simulink model "motor_simulink"  (R2021b)
settings: Solver=VariableStepAuto  StartTime=0.0  StopTime=1.5  MaxStep=1e-8  RelTol=1e-3
libraries: simulink x7, spsOnDelayLib x6, slpidlib x3, eePwmGeneratorTwoLevel x2, spsDCVoltageSourceLib x1, spsPermanentMagnetSynchronousMachineLib x1, spsUniversalBridgeLib x1, spsabctodq0Lib x1, spspowerguiLib x1
settings Model: SimulationMode=accelerator  Creator=phddk  LastModifiedBy=phddk
settings SolverCC: ZeroCrossAlgorithm=Adaptive

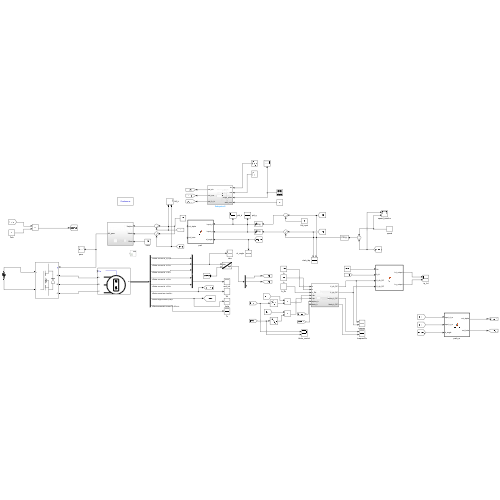
[thumbnail: Simulink's stored preview of the top-level diagram]
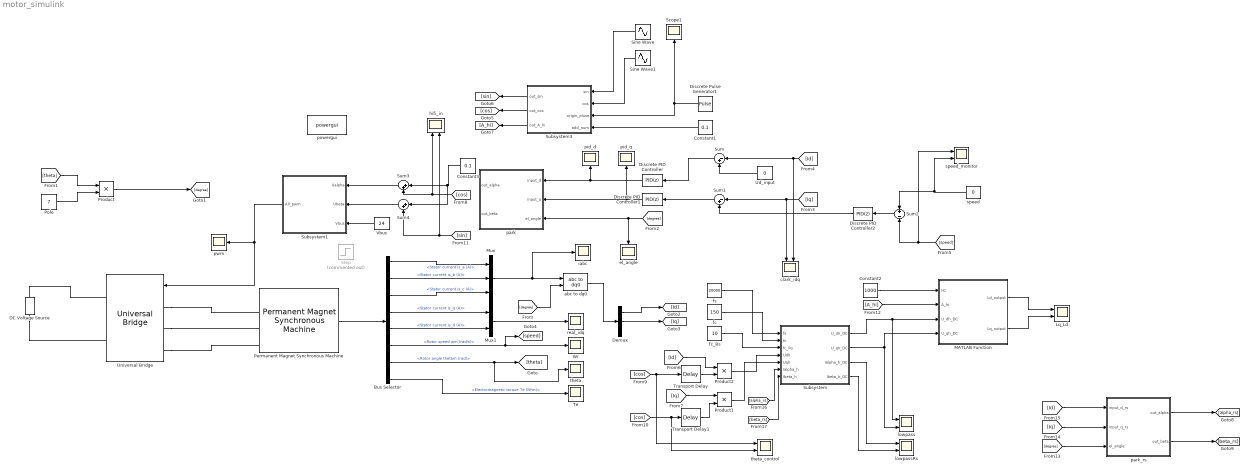
== system motor_simulink ==
  Bus Selector : BusSelector  OutputSignals=Stator current is_a (A),Stator current is_b (A),Stator current is_c (A),Stator current is_q (A),Stator current is_d (A),Rotor speed wm (rad/s),Rotor angle thetam (rad),Electromagnetic torque Te (N*m)
  Constant1 : Constant  Value=0.1
  Constant2 : Constant  Value=1000
  Constant3 : Constant  Value=0.1
  DC Voltage Source : spsDCVoltageSourceLib/DC Voltage Source  Amplitude=24  Measurements=Voltage
  Demux : Demux  Outputs=3
  Discrete Pulse Generator1 : DiscretePulseGenerator  Period=50  PulseWidth=25  SampleTime=0.001
  Discrete PID Controller : slpidlib/PID Controller  Controller=PID  Form=Parallel  TimeDomain=Discrete-time  UseExternalTs=off  SampleTime=-1  IntegratorMethod=Forward Euler  FilterMethod=Forward Euler  ControllerParametersSource=internal  P=1  I=5  D=0  UseFilter=on  N=100  TunerSelectOption=Transfer Function Based (PID Tuner App)  InitialConditionSource=internal  InitialConditionForIntegrator=0  InitialConditionForFilter=0  DifferentiatorICPrevScaledInput=0  ExternalReset=none  TrackingMode=off  Kt=1  LimitOutput=on  SatLimitsSource=internal  UpperSaturationLimit=24  LowerSaturationLimit=-24  LinearizeAsGain=off  AntiWindupMode=none  Kb=1  POutMin=[]  POutMax=[]  IOutMin=[-20]  IOutMax=[20]  DOutMin=[]  DOutMax=[]  NOutMin=[]  NOutMax=[]  SumOutMin=[]  SumOutMax=[]  SaturationOutMin=[]  SaturationOutMax=[]  PParamMin=[]  PParamMax=[]  IParamMin=[]  IParamMax=[]  DParamMin=[]  DParamMax=[]  NParamMin=[]  NParamMax=[]  KbParamMin=[]  KbParamMax=[]  KtParamMin=[]  KtParamMax=[]  KbOutMin=[]  KbOutMax=[]  KtOutMin=[]  KtOutMax=[]  IntegratorOutMin=[]  IntegratorOutMax=[]  FilterOutMin=[]  FilterOutMax=[]  SumI1OutMin=[]  SumI1OutMax=[]  SumI2OutMin=[]  SumI2OutMax=[]  SumI3OutMin=[]  SumI3OutMax=[]  SumI4OutMin=[]  SumI4OutMax=[]  SumDOutMin=[]  SumDOutMax=[]  DifferentiatorOutMin=[]  DifferentiatorOutMax=[]  FilterDiffOutCoefMin=[]  FilterDiffOutCoefMax=[]  ReciprocalOutMin=[]  ReciprocalOutMax=[]  SumDenOutMin=[]  SumDenOutMax=[]  SumNumOutMin=[]  SumNumOutMax=[]  DivideOutMin=[]  DivideOutMax=[]  UdiffTsProdOutMin=[]  UdiffTsProdOutMax=[]  NTsProdOutMin=[]  NTsProdOutMax=[]  UintegralTsProdOutMin=[]  UintegralTsProdOutMax=[]  UngainTsProdOutMin=[]  UngainTsProdOutMax=[]  IntegratorContinuousStateAttributes=''  IntegratorStateMustResolveToSignalObject=off  IntegratorRTWStateStorageClass=Auto  FilterContinuousStateAttributes=''  FilterStateMustResolveToSignalObject=off  FilterRTWStateStorageClass=Auto  ParallelPVariant=InternalParameters  IdealPVariant=Disabled  IVariant=InternalParameters  DVariant=InternalParameters  IntegratorVariant=Discrete  SatVariant=Enabled  AWVariant=Passthrough  PCopyVariant=Disabled  TRVariant=Disabled  FdbkBlocksVariant=Forward  IdealPFdbkVariant=Disabled  SatFdbkVariant=Disabled  DerivativeFilterVariant=ForwardEulerFilter  NVariant=InternalParameters  NCopyVariant=Disabled  FilterICVariant=InternalICsFilter  IntegratorICVariant=InternalICs  ExternalResetVariant=Disabled  TRSumVariant=Passthrough  SumFdbkVariant=Disabled  SumVariant=Sum_PID  TsampFilterVariant=InternalTs  TsampNgainVariant=Passthrough  TsampIntegralVariant=Passthrough  ExternalSaturationOutDataTypeStr=Inherit: Same as second input
  Discrete PID Controller1 : slpidlib/PID Controller  Controller=PID  Form=Parallel  TimeDomain=Discrete-time  UseExternalTs=off  SampleTime=-1  IntegratorMethod=Forward Euler  FilterMethod=Forward Euler  ControllerParametersSource=internal  P=1  I=5  D=0  UseFilter=on  N=100  TunerSelectOption=Transfer Function Based (PID Tuner App)  InitialConditionSource=internal  InitialConditionForIntegrator=0  InitialConditionForFilter=0  DifferentiatorICPrevScaledInput=0  ExternalReset=none  TrackingMode=off  Kt=1  LimitOutput=on  SatLimitsSource=internal  UpperSaturationLimit=24  LowerSaturationLimit=-24  LinearizeAsGain=off  AntiWindupMode=none  Kb=1  POutMin=[]  POutMax=[]  IOutMin=[-20]  IOutMax=[20]  DOutMin=[]  DOutMax=[]  NOutMin=[]  NOutMax=[]  SumOutMin=[]  SumOutMax=[]  SaturationOutMin=[]  SaturationOutMax=[]  PParamMin=[]  PParamMax=[]  IParamMin=[]  IParamMax=[]  DParamMin=[]  DParamMax=[]  NParamMin=[]  NParamMax=[]  KbParamMin=[]  KbParamMax=[]  KtParamMin=[]  KtParamMax=[]  KbOutMin=[]  KbOutMax=[]  KtOutMin=[]  KtOutMax=[]  IntegratorOutMin=[]  IntegratorOutMax=[]  FilterOutMin=[]  FilterOutMax=[]  SumI1OutMin=[]  SumI1OutMax=[]  SumI2OutMin=[]  SumI2OutMax=[]  SumI3OutMin=[]  SumI3OutMax=[]  SumI4OutMin=[]  SumI4OutMax=[]  SumDOutMin=[]  SumDOutMax=[]  DifferentiatorOutMin=[]  DifferentiatorOutMax=[]  FilterDiffOutCoefMin=[]  FilterDiffOutCoefMax=[]  ReciprocalOutMin=[]  ReciprocalOutMax=[]  SumDenOutMin=[]  SumDenOutMax=[]  SumNumOutMin=[]  SumNumOutMax=[]  DivideOutMin=[]  DivideOutMax=[]  UdiffTsProdOutMin=[]  UdiffTsProdOutMax=[]  NTsProdOutMin=[]  NTsProdOutMax=[]  UintegralTsProdOutMin=[]  UintegralTsProdOutMax=[]  UngainTsProdOutMin=[]  UngainTsProdOutMax=[]  IntegratorContinuousStateAttributes=''  IntegratorStateMustResolveToSignalObject=off  IntegratorRTWStateStorageClass=Auto  FilterContinuousStateAttributes=''  FilterStateMustResolveToSignalObject=off  FilterRTWStateStorageClass=Auto  ParallelPVariant=InternalParameters  IdealPVariant=Disabled  IVariant=InternalParameters  DVariant=InternalParameters  IntegratorVariant=Discrete  SatVariant=Enabled  AWVariant=Passthrough  PCopyVariant=Disabled  TRVariant=Disabled  FdbkBlocksVariant=Forward  IdealPFdbkVariant=Disabled  SatFdbkVariant=Disabled  DerivativeFilterVariant=ForwardEulerFilter  NVariant=InternalParameters  NCopyVariant=Disabled  FilterICVariant=InternalICsFilter  IntegratorICVariant=InternalICs  ExternalResetVariant=Disabled  TRSumVariant=Passthrough  SumFdbkVariant=Disabled  SumVariant=Sum_PID  TsampFilterVariant=InternalTs  TsampNgainVariant=Passthrough  TsampIntegralVariant=Passthrough  ExternalSaturationOutDataTypeStr=Inherit: Same as second input
  Discrete PID Controller2 : slpidlib/PID Controller  Controller=PID  Form=Parallel  TimeDomain=Discrete-time  UseExternalTs=off  SampleTime=-1  IntegratorMethod=Forward Euler  FilterMethod=Forward Euler  ControllerParametersSource=internal  P=2  I=0  D=0  UseFilter=on  N=100  TunerSelectOption=Transfer Function Based (PID Tuner App)  InitialConditionSource=internal  InitialConditionForIntegrator=0  InitialConditionForFilter=0  DifferentiatorICPrevScaledInput=0  ExternalReset=none  TrackingMode=off  Kt=1  LimitOutput=off  SatLimitsSource=internal  UpperSaturationLimit=24  LowerSaturationLimit=-24  LinearizeAsGain=off  AntiWindupMode=none  Kb=1  POutMin=[]  POutMax=[]  IOutMin=[]  IOutMax=[]  DOutMin=[]  DOutMax=[]  NOutMin=[]  NOutMax=[]  SumOutMin=[]  SumOutMax=[]  SaturationOutMin=[]  SaturationOutMax=[]  PParamMin=[]  PParamMax=[]  IParamMin=[]  IParamMax=[]  DParamMin=[]  DParamMax=[]  NParamMin=[]  NParamMax=[]  KbParamMin=[]  KbParamMax=[]  KtParamMin=[]  KtParamMax=[]  KbOutMin=[]  KbOutMax=[]  KtOutMin=[]  KtOutMax=[]  IntegratorOutMin=[]  IntegratorOutMax=[]  FilterOutMin=[]  FilterOutMax=[]  SumI1OutMin=[]  SumI1OutMax=[]  SumI2OutMin=[]  SumI2OutMax=[]  SumI3OutMin=[]  SumI3OutMax=[]  SumI4OutMin=[]  SumI4OutMax=[]  SumDOutMin=[]  SumDOutMax=[]  DifferentiatorOutMin=[]  DifferentiatorOutMax=[]  FilterDiffOutCoefMin=[]  FilterDiffOutCoefMax=[]  ReciprocalOutMin=[]  ReciprocalOutMax=[]  SumDenOutMin=[]  SumDenOutMax=[]  SumNumOutMin=[]  SumNumOutMax=[]  DivideOutMin=[]  DivideOutMax=[]  UdiffTsProdOutMin=[]  UdiffTsProdOutMax=[]  NTsProdOutMin=[]  NTsProdOutMax=[]  UintegralTsProdOutMin=[]  UintegralTsProdOutMax=[]  UngainTsProdOutMin=[]  UngainTsProdOutMax=[]  IntegratorContinuousStateAttributes=''  IntegratorStateMustResolveToSignalObject=off  IntegratorRTWStateStorageClass=Auto  FilterContinuousStateAttributes=''  FilterStateMustResolveToSignalObject=off  FilterRTWStateStorageClass=Auto  ParallelPVariant=InternalParameters  IdealPVariant=Disabled  IVariant=InternalParameters  DVariant=InternalParameters  IntegratorVariant=Discrete  SatVariant=Disabled  AWVariant=Passthrough  PCopyVariant=Disabled  TRVariant=Disabled  FdbkBlocksVariant=Forward  IdealPFdbkVariant=Disabled  SatFdbkVariant=Disabled  DerivativeFilterVariant=ForwardEulerFilter  NVariant=InternalParameters  NCopyVariant=Disabled  FilterICVariant=InternalICsFilter  IntegratorICVariant=InternalICs  ExternalResetVariant=Disabled  TRSumVariant=Passthrough  SumFdbkVariant=Disabled  SumVariant=Sum_PID  TsampFilterVariant=InternalTs  TsampNgainVariant=Passthrough  TsampIntegralVariant=Passthrough  ExternalSaturationOutDataTypeStr=Inherit: Same as second input
  Lq_Ld : Scope  NumInputPorts=2
  MATLAB Function : MATLAB Function  TreatAsAtomicUnit=on
  Mux : Mux  Inputs=3
  Mux1 : Mux  Inputs=2
  Permanent Magnet Synchronous Machine : spsPermanentMagnetSynchronousMachineLib/Permanent Magnet Synchronous Machine  NbPhases=3  FluxDistribution=Sinusoidal  RotorType=Round  MechanicalLoad=Torque Tm  PresetModel=No  ShowDetailedParameters=on  MeasurementBus=off  Resistance=0.1  Inductance=8.5e-3  dqInductances=[8.5e-3,8.5e-3]  La=1E-3  MachineConstant=Flux linkage established by magnets (V.s)  Flux=0.00185  VoltageCst=2.3489  TorqueCst=0.019425  Flat=120  Mechanical=[0.0027 0.0004924 7 0]  PolePairs=4  InitialConditions=[0,0, 0,0]  InitialConditions5ph=[0 0 0 0 0 0]  RefAngle=Aligned with phase A axis (original Park)  IterativeDiscreteModel=Trapezoidal non iterative  TsBlock=-1  TsPowergui=0
  Pole : Constant  Value=7
  Product : Product
  Product1 : Product
  Product2 : Product
  Scope1 : Scope
  Sine Wave : Sin  SineType=Sample based  Amplitude=0.3  Frequency=1000  Samples=126  SampleTime=5e-5
  Sine Wave1 : Sin  SineType=Sample based  Amplitude=0.3  Frequency=1000  Phase=0.5*pi  Samples=126  SampleTime=5e-5  Offset=32
  Step : Step  Commented=on  Time=0.35  After=0  SampleTime=0
  Subsystem : Subsystem
  Subsystem1 : Subsystem
  Subsystem3 : Subsystem
  Sum : Sum  Inputs=|-+
  Sum1 : Sum  Inputs=|-+
  Sum2 : Sum  Inputs=+-
  Sum3 : Sum  Inputs=|++
  Sum4 : Sum  Inputs=|++
  Te : Scope
  Transport Delay : TransportDelay  DelayTime=2e-8
  Transport Delay1 : TransportDelay  DelayTime=2e-8
  Ud_input : Constant  Value=0
  Universal Bridge : spsUniversalBridgeLib/Universal Bridge  Arms=3  SnubberResistance=1e5  SnubberCapacitance=inf  Device=MOSFET / Diodes  Ron=1e-3  Lon=0  ForwardVoltages="[  0  0  ]"  ForwardVoltage=0  GTOparameters=[ 10e-6 , 20e-6 ]  IGBTparameters=[ 1e-6 , 2e-6 ]  Measurements=None  Measurements_2=None  converterType=Rectifier
  Vbus : Constant  Value=24
  Wr : Scope
  abc to dq0 : spsabctodq0Lib/abc to dq0  Alignment=Aligned with phase A axis
  clark_idq : Scope  NumInputPorts=2
  el_angle : Scope
  fc : Constant  Value=150
  fc_Rs : Constant  Value=10
  fs : Constant  Value=20000
  hifi_in : Scope  NumInputPorts=2
  iabc : Scope
  lowpass : Scope  NumInputPorts=2
  lowpassRs : Scope  NumInputPorts=2
  park : MATLAB Function  TreatAsAtomicUnit=on
  park_rs : MATLAB Function  TreatAsAtomicUnit=on
  pid_d : Scope
  pid_q : Scope
  powergui : spspowerguiLib/powergui  Priority=1  SimulationMode=Continuous  SampleTime=1e-5  frequency=60  Iterations=50  frequencyindice=0  Pbase=100e6  ErrMax=1e-4  UnitsV=kV  UnitsW=MW  buscounter=0  FunctionMessages=off  echomessages=off  EnableUseOfTLC=off  CurrentSourceSwitches=off  DisableSnubberDevices=off  DisableRonSwitches=off  DisableVfSwitches=off  DisplayEquations=off  AutomaticDiscreteSolvers=off  SolverType=Tustin/Backward Euler (TBE)  Interpol=off  ExternalGateDelay=off  methode=off  Ts=100  x0status=blocks  SPID=on  SwTol=0  HookPort=off  NonlinearTolerance=1e-4  nMaxIteration=100  ContinueOnMaxIteration=off  RestoreLinks=warning  ResistiveCurrentMeasurement=off  Frange=[0:2:500]  Ylog=off  Xlog=on  ShowGrid=off  save=off  variable=ZData  structure=0  ZoomFFT=off  StartTime=0.0  cycles=1  DisplayStyle=1  fundamental=60  FreqAxis=off  MaxFrequency=1000  frequencyindicesteady=1  RmsSteady=1  display=off
  pwm : Scope
  real_idq : Scope
  speed : Constant  Value=0
  speed_monitor : Scope  NumInputPorts=2
  theta : Scope
  theta_control : Scope  NumInputPorts=2
  wires:
  Permanent Magnet Synchronous Machine/1 -> Bus Selector/1
  Bus Selector/1 -> Mux/1  "<Stator current is_a (A)>"
  Bus Selector/2 -> Mux/2  "<Stator current is_b (A)>"
  Bus Selector/3 -> Mux/3  "<Stator current is_c (A)>"
  Bus Selector/4 -> Mux1/1  "<Stator current is_q (A)>"
  Bus Selector/5 -> Mux1/2  "<Stator current is_d (A)>"
  Bus Selector/7 -> theta/1, [theta]  "<Rotor angle thetam (rad)>"
  Bus Selector/8 -> Te/1  "<Electromagnetic torque Te (N*m)>"
  Mux/1 -> iabc/1, abc to dq0/1
  [degree] -> abc to dq0/2
  Pole/1 -> Product/2
  [theta] -> Product/1
  abc to dq0/1 -> Demux/1
  Demux/1 -> [Id]
  Demux/2 -> [Iq]
  Mux1/1 -> real_idq/1
  Subsystem1/1(All_pwm) -> Universal Bridge/1, pwm/1
  Vbus/1 -> Subsystem1/3(Vbus)
  [degree] -> el_angle/1, park/3(el_angle)
  [Id] -> clark_idq/2, Sum/1
  [Iq] -> Sum1/1, clark_idq/1
  Sum/1 -> Discrete PID Controller/1
  Sum1/1 -> Discrete PID Controller1/1
  Discrete PID Controller/1 -> park/1(input_d), pid_d/1
  Product/1 -> [degree]
  Bus Selector/6 -> Wr/1, [speed]  "<Rotor speed wm (rad/s)>"
  [speed] -> speed_monitor/1, Sum2/2
  speed/1 -> speed_monitor/2, Sum2/1
  Sum2/1 -> Discrete PID Controller2/1
  Discrete PID Controller1/1 -> pid_q/1, park/2(input_q)
  Ud_input/1 -> Sum/2
  Discrete PID Controller2/1 -> Sum1/2
  fs/1 -> Subsystem/1(fs)
  fc/1 -> Subsystem/2(fc)
  Sum4/1 -> Subsystem1/2(Ubeta)
  Sum3/1 -> Subsystem1/1(Ualpha)
  [Id] -> Product2/1
  Product2/1 -> Subsystem/4(Udh)
  [Iq] -> Product1/1
  Product1/1 -> Subsystem/5(Uqh)
  [cos] -> theta_control/2, Transport Delay1/1
  [cos] -> theta_control/1, Transport Delay/1
  Discrete Pulse Generator1/1 -> Subsystem3/3(origin_pluse), Scope1/1
  Constant1/1 -> Subsystem3/4(add_num)
  [cos] -> hifi_in/1, Sum3/2
  [sin] -> hifi_in/2, Sum4/2
  Constant2/1 -> MATLAB Function/1(Hz)
  [A_hi] -> MATLAB Function/2(A_hi)
  Subsystem/2(U_qh_DC) -> lowpass/2, MATLAB Function/4(U_qh_DC)
  MATLAB Function/1(Ld_output) -> Lq_Ld/1
  MATLAB Function/2(Lq_output) -> Lq_Ld/2
  Transport Delay/1 -> Product2/2
  Transport Delay1/1 -> Product1/2
  fc_Rs/1 -> Subsystem/3(fc_Rs)
  [degree] -> park_rs/3(el_angle)
  [Iq] -> park_rs/2(input_q_rs)
  [Id] -> park_rs/1(input_d_rs)
  park_rs/1(out_alpha) -> [alpha_rs]
  park_rs/2(out_beta) -> [beta_rs]
  [alpha_rs] -> Subsystem/6(Ialpha_h)
  [beta_rs] -> Subsystem/7(Ibeta_h)
  Subsystem/1(U_dh_DC) -> MATLAB Function/3(U_dh_DC), lowpass/1
  Subsystem/3(Ialpha_h_DC) -> lowpassRs/1
  Subsystem/4(Ibeta_h_DC) -> lowpassRs/2
  Subsystem3/1(out_sin) -> [sin]
  Subsystem3/2(out_cos) -> [cos]
  Subsystem3/3(out_A_hi) -> [A_hi]
  Sine Wave/1 -> Subsystem3/1(sin)
  Sine Wave1/1 -> Subsystem3/2(cos)
  Constant3/1 -> Sum4/1, Sum3/1
  connections:
  DC Voltage Source/RConn1 -- Universal Bridge/RConn1
  DC Voltage Source/LConn1 -- Universal Bridge/RConn2
  Universal Bridge/LConn1 -- Permanent Magnet Synchronous Machine/LConn1
  Universal Bridge/LConn2 -- Permanent Magnet Synchronous Machine/LConn2
  Universal Bridge/LConn3 -- Permanent Magnet Synchronous Machine/LConn3

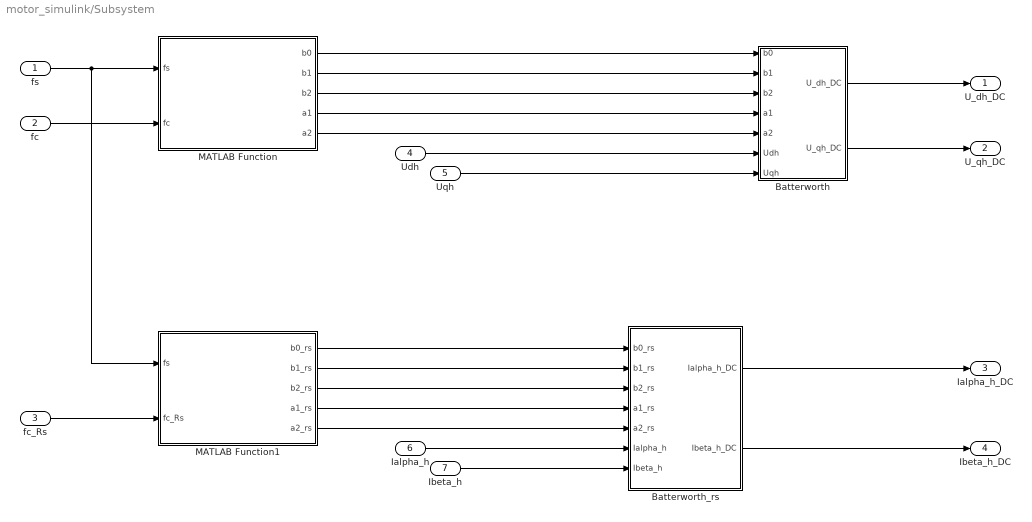
== system motor_simulink/Subsystem ==
  fs : Inport
  fc : Inport  Port=2
  fc_Rs : Inport  Port=3
  Udh : Inport  Port=4
  Uqh : Inport  Port=5
  Ialpha_h : Inport  Port=6
  Ibeta_h : Inport  Port=7
  Batterworth : MATLAB Function  TreatAsAtomicUnit=on  SystemSampleTime=0.0001
  Batterworth_rs : MATLAB Function  TreatAsAtomicUnit=on  SystemSampleTime=0.0001
  MATLAB Function : MATLAB Function  TreatAsAtomicUnit=on
  MATLAB Function1 : MATLAB Function  TreatAsAtomicUnit=on
  U_dh_DC : Outport
  U_qh_DC : Outport  Port=2
  Ialpha_h_DC : Outport  Port=3
  Ibeta_h_DC : Outport  Port=4
  wires:
  Uqh/1 -> Batterworth/7(Uqh)
  fs/1 -> MATLAB Function1/1(fs), MATLAB Function/1(fs)
  MATLAB Function/4(a1) -> Batterworth/4(a1)
  MATLAB Function/1(b0) -> Batterworth/1(b0)
  MATLAB Function/5(a2) -> Batterworth/5(a2)
  MATLAB Function/3(b2) -> Batterworth/3(b2)
  MATLAB Function/2(b1) -> Batterworth/2(b1)
  Udh/1 -> Batterworth/6(Udh)
  Batterworth/2(U_qh_DC) -> U_qh_DC/1
  Batterworth/1(U_dh_DC) -> U_dh_DC/1
  fc/1 -> MATLAB Function/2(fc)
  fc_Rs/1 -> MATLAB Function1/2(fc_Rs)
  MATLAB Function1/1(b0_rs) -> Batterworth_rs/1(b0_rs)
  MATLAB Function1/2(b1_rs) -> Batterworth_rs/2(b1_rs)
  MATLAB Function1/3(b2_rs) -> Batterworth_rs/3(b2_rs)
  MATLAB Function1/4(a1_rs) -> Batterworth_rs/4(a1_rs)
  MATLAB Function1/5(a2_rs) -> Batterworth_rs/5(a2_rs)
  Ialpha_h/1 -> Batterworth_rs/6(Ialpha_h)
  Batterworth_rs/1(Ialpha_h_DC) -> Ialpha_h_DC/1
  Batterworth_rs/2(Ibeta_h_DC) -> Ibeta_h_DC/1
  Ibeta_h/1 -> Batterworth_rs/7(Ibeta_h)

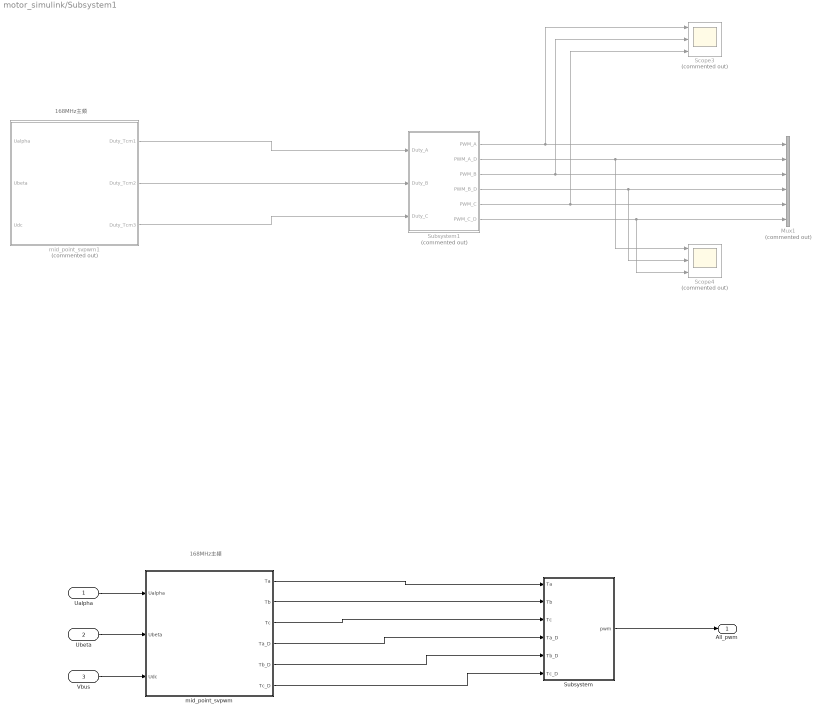
== system motor_simulink/Subsystem1 ==
  note: 168MHz主频
  note: 168MHz主频
  Ualpha : Inport
  Ubeta : Inport  Port=2
  Vbus : Inport  Port=3
  Mux1 : Mux  Commented=on  Inputs=6
  Scope3 : Scope  Commented=on  NumInputPorts=3
  Scope4 : Scope  Commented=on  NumInputPorts=3
  Subsystem : Subsystem
  Subsystem1 : Subsystem  Commented=on
  mid_point_svpwm : MATLAB Function  TreatAsAtomicUnit=on
  mid_point_svpwm1 : MATLAB Function  Commented=on  TreatAsAtomicUnit=on
  All_pwm : Outport
  wires:
  mid_point_svpwm/1(Ta) -> Subsystem/1(Ta)
  mid_point_svpwm/3(Tc) -> Subsystem/3(Tc)
  Ualpha/1 -> mid_point_svpwm/1(Ualpha)
  Ubeta/1 -> mid_point_svpwm/2(Ubeta)
  Vbus/1 -> mid_point_svpwm/3(Udc)
  Subsystem1/1(PWM_A) -> Scope3/1, Mux1/1
  mid_point_svpwm1/3(Duty_Tcm3) -> Subsystem1/3(Duty_C)
  Subsystem1/6(PWM_C_D) -> Scope4/3, Mux1/6
  Subsystem1/5(PWM_C) -> Scope3/3, Mux1/5
  mid_point_svpwm1/2(Duty_Tcm2) -> Subsystem1/2(Duty_B)
  Subsystem1/4(PWM_B_D) -> Scope4/2, Mux1/4
  mid_point_svpwm1/1(Duty_Tcm1) -> Subsystem1/1(Duty_A)
  Subsystem1/3(PWM_B) -> Scope3/2, Mux1/3
  Subsystem1/2(PWM_A_D) -> Scope4/1, Mux1/2
  Subsystem/1(pwm) -> All_pwm/1
  mid_point_svpwm/2(Tb) -> Subsystem/2(Tb)
  mid_point_svpwm/4(Ta_D) -> Subsystem/4(Ta_D)
  mid_point_svpwm/5(Tb_D) -> Subsystem/5(Tb_D)
  mid_point_svpwm/6(Tc_D) -> Subsystem/6(Tc_D)

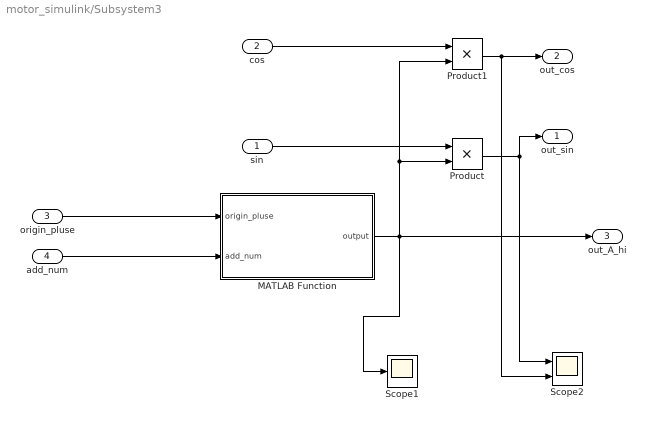
== system motor_simulink/Subsystem3 ==
  sin : Inport
  cos : Inport  Port=2
  origin_pluse : Inport  Port=3
  add_num : Inport  Port=4
  MATLAB Function : MATLAB Function  TreatAsAtomicUnit=on
  Product : Product
  Product1 : Product
  Scope1 : Scope
  Scope2 : Scope  NumInputPorts=2
  out_sin : Outport
  out_cos : Outport  Port=2
  out_A_hi : Outport  Port=3
  wires:
  MATLAB Function/1(output) -> Product1/2, Product/2, out_A_hi/1, Scope1/1
  sin/1 -> Product/1
  Product/1 -> out_sin/1, Scope2/1
  add_num/1 -> MATLAB Function/2(add_num)
  origin_pluse/1 -> MATLAB Function/1(origin_pluse)
  cos/1 -> Product1/1
  Product1/1 -> Scope2/2, out_cos/1

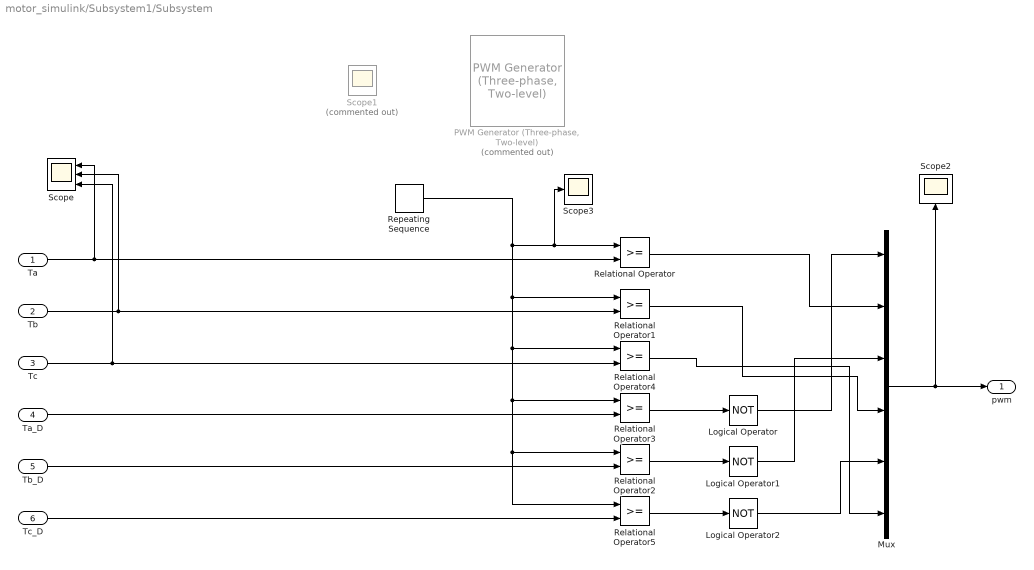
== system motor_simulink/Subsystem1/Subsystem ==
  Ta : Inport  OutDataTypeStr=double
  Tb : Inport  Port=2  OutDataTypeStr=double
  Tc : Inport  Port=3  OutDataTypeStr=double
  Ta_D : Inport  Port=4  OutDataTypeStr=double
  Tb_D : Inport  Port=5  OutDataTypeStr=double
  Tc_D : Inport  Port=6  OutDataTypeStr=double
  Logical Operator : Logic  Operator=NOT  AllPortsSameDT=off  OutDataTypeStr=boolean
  Logical Operator1 : Logic  Operator=NOT  AllPortsSameDT=off  OutDataTypeStr=boolean
  Logical Operator2 : Logic  Operator=NOT  AllPortsSameDT=off  OutDataTypeStr=boolean
  Mux : Mux  Inputs=6
  "PWM Generator (Three-phase, Two-level)" : eePwmGeneratorTwoLevel/PWM Generator (Three-phase, Two-level)  Commented=on  PWMMode=Continuous PWM (CPWM)  CPWMMode=SPWM: sinusoidal PWM  DPWMMode=60 DPWM: 60 degree discontinuous PWM  fsw=20000  Ts=0.000005
      settings: SourceProductBaseCode=PS
  Relational Operator{,1..5} (6 alike) : RelationalOperator  OutDataTypeStr=boolean  RndMeth=Simplest
  Repeating Sequence : simulink/Sources/Repeating Sequence  rep_seq_t=[0, 2.5e-5, 5e-5]  rep_seq_y=[0,2880,0]
  Scope : Scope  NumInputPorts=3
  Scope1 : Scope  Commented=on
  Scope2 : Scope
  Scope3 : Scope
  pwm : Outport
  wires:
  Relational Operator3/1 -> Logical Operator/1
  Repeating Sequence/1 -> Relational Operator5/1, Relational Operator2/1, Relational Operator3/1, Relational Operator4/1, Relational Operator1/1, Scope3/1, Relational Operator/1
  Relational Operator2/1 -> Logical Operator1/1
  Relational Operator5/1 -> Logical Operator2/1
  Tb/1 -> Scope/2, Relational Operator1/2
  Tc/1 -> Scope/3, Relational Operator4/2
  Mux/1 -> pwm/1, Scope2/1
  Ta/1 -> Relational Operator/2, Scope/1
  Ta_D/1 -> Relational Operator3/2
  Tb_D/1 -> Relational Operator2/2
  Tc_D/1 -> Relational Operator5/2
  Relational Operator/1 -> Mux/2
  Logical Operator/1 -> Mux/1
  Logical Operator1/1 -> Mux/3
  Relational Operator1/1 -> Mux/4
  Logical Operator2/1 -> Mux/5
  Relational Operator4/1 -> Mux/6

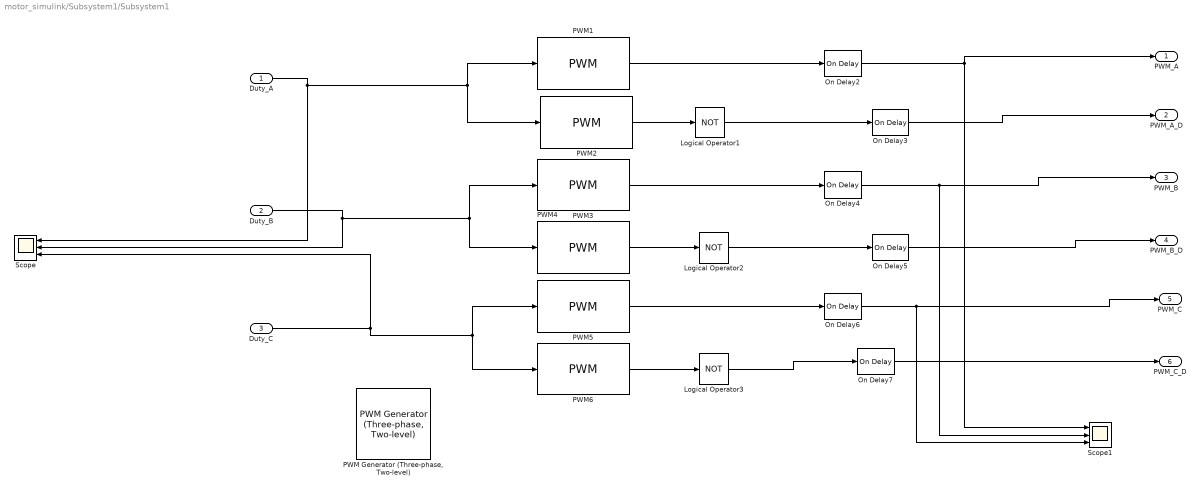
== system motor_simulink/Subsystem1/Subsystem1 ==
  Duty_A : Inport  OutDataTypeStr=double
  Duty_B : Inport  Port=2  OutDataTypeStr=double
  Duty_C : Inport  Port=3  OutDataTypeStr=double
  Logical Operator1 : Logic  Operator=NOT  AllPortsSameDT=off  OutDataTypeStr=boolean
  Logical Operator2 : Logic  Operator=NOT  AllPortsSameDT=off  OutDataTypeStr=boolean
  Logical Operator3 : Logic  Operator=NOT  AllPortsSameDT=off  OutDataTypeStr=boolean
  On Delay{2..7} (6 alike) : spsOnDelayLib/On Delay  DelayType=On delay  delay=5e-6  ic=0  Ts=0
      settings: SourceProductBaseCode=PS
  "PWM Generator (Three-phase, Two-level)" : eePwmGeneratorTwoLevel/PWM Generator (Three-phase, Two-level)  PWMMode=Continuous PWM (CPWM)  CPWMMode=SPWM: sinusoidal PWM  DPWMMode=60 DPWM: 60 degree discontinuous PWM  fsw=2000  Ts=5e-5
      settings: SourceProductBaseCode=PS
  PWM{1..6} (6 alike) : simulink/Discontinuities/PWM  DisableCoverage=on  Period=5e-4  DisallowZeroDutyCycle=off  RunAtFixedTimeIntervals=on  SampleTime=5e-5
  Scope : Scope  NumInputPorts=3
  Scope1 : Scope  NumInputPorts=3
  PWM_A : Outport  OutDataTypeStr=double
  PWM_A_D : Outport  Port=2  OutDataTypeStr=double
  PWM_B : Outport  Port=3  OutDataTypeStr=double
  PWM_B_D : Outport  Port=4  OutDataTypeStr=double
  PWM_C : Outport  Port=5  OutDataTypeStr=double
  PWM_C_D : Outport  Port=6  OutDataTypeStr=double
  wires:
  PWM4/1 -> Logical Operator2/1
  PWM6/1 -> Logical Operator3/1
  PWM2/1 -> Logical Operator1/1
  PWM3/1 -> On Delay4/1
  PWM1/1 -> On Delay2/1
  On Delay2/1 -> PWM_A/1, Scope1/1
  Duty_A/1 -> PWM2/1, PWM1/1, Scope/1
  PWM5/1 -> On Delay6/1
  On Delay3/1 -> PWM_A_D/1
  On Delay4/1 -> Scope1/2, PWM_B/1
  On Delay5/1 -> PWM_B_D/1
  On Delay6/1 -> Scope1/3, PWM_C/1
  On Delay7/1 -> PWM_C_D/1
  Duty_B/1 -> PWM4/1, PWM3/1, Scope/2
  Duty_C/1 -> PWM5/1, PWM6/1, Scope/3
  Logical Operator1/1 -> On Delay3/1
  Logical Operator3/1 -> On Delay7/1
  Logical Operator2/1 -> On Delay5/1

== matlab function motor_simulink/Subsystem/MATLAB Function1 ==
  data: fs input; b0_rs output; fc_Rs input; b1_rs output; b2_rs output; a1_rs output; a2_rs output
function [b0_rs, b1_rs, b2_rs, a1_rs, a2_rs] = butterworth_2nd_Rs(fs, fc_Rs)

persistent first_flag_rs
persistent b_0_rs
persistent b_1_rs
persistent b_2_rs
persistent a_1_rs
persistent a_2_rs

if isempty(first_flag_rs)

    Wn_rs = fc_Rs / (fs/2);

    [b_rs, a_rs] = butter(2, Wn_rs, 'low');

    b_0_rs = b_rs(1);
    b_1_rs = b_rs(2);
    b_2_rs = b_rs(3);

    a_1_rs = a_rs(2);
    a_2_rs = a_rs(3);

    first_flag_rs=true;
end

b0_rs = b_0_rs;
b1_rs = b_1_rs;
b2_rs = b_2_rs;

a1_rs = a_1_rs;
a2_rs = a_2_rs;

end

== matlab function motor_simulink/Subsystem/Batterworth_rs ==
  data: b0_rs input; Ialpha_h_DC output; b1_rs input; b2_rs input; a1_rs input; a2_rs input; Ibeta_h_DC output; Ialpha_h input; Ibeta_h input
function [Ialpha_h_DC,Ibeta_h_DC]= fcn_rs(b0_rs,b1_rs,b2_rs,a1_rs,a2_rs,Ialpha_h,Ibeta_h)

persistent first_flag_rs
persistent x_0_rs
persistent x_1_rs
persistent x_2_rs
persistent x_3_rs
persistent x_4_rs
persistent x_5_rs
persistent y_1_rs
persistent y_2_rs
persistent y_3_rs
persistent y_4_rs
persistent y_0_alpha
persistent y_0_beta
if isempty(first_flag_rs)
    Ialpha_h_DC=0;
    Ibeta_h_DC=0;
    x_0_rs=0;
    x_1_rs=0;
    x_2_rs=0;
    y_1_rs=0;
    y_2_rs=0;
    x_3_rs=0;
    x_4_rs=0;
    x_5_rs=0;
    y_3_rs=0;
    y_4_rs=0;
    y_0_alpha=0;
    y_0_beta=0;

    first_flag_rs=true;
end

x_2_rs = x_1_rs;
x_1_rs = x_0_rs;
x_0_rs = Ialpha_h;

x_5_rs = x_4_rs;
x_4_rs = x_3_rs;
x_3_rs = Ibeta_h;

y_2_rs = y_1_rs;
y_1_rs = y_0_alpha;

y_4_rs = y_3_rs;
y_3_rs = y_0_beta;


Ialpha_h_DC = b0_rs*x_0_rs + b1_rs*x_1_rs + b2_rs*x_2_rs - a1_rs*y_1_rs - a2_rs*y_2_rs;
Ibeta_h_DC = b0_rs*x_3_rs + b1_rs*x_4_rs + b2_rs*x_5_rs - a1_rs*y_3_rs - a2_rs*y_4_rs;

y_0_alpha = Ialpha_h_DC;
y_0_beta = Ibeta_h_DC;

end

== matlab function motor_simulink/park_rs ==
  data: input_d_rs input; out_alpha output; input_q_rs input; out_beta output; el_angle input
function [out_alpha, out_beta] = park_rs(input_d_rs, input_q_rs, el_angle)

out_alpha =( input_d_rs * cos(el_angle) - input_q_rs * sin(el_angle));
out_beta = (input_d_rs * sin(el_angle) + input_q_rs * cos(el_angle));

end

== matlab function motor_simulink/park ==
  data: input_d input; out_alpha output; input_q input; out_beta output; el_angle input
function [out_alpha, out_beta] = fcn(input_d, input_q, el_angle)

out_alpha =( input_d * cos(el_angle) - input_q * sin(el_angle));
out_beta = (input_d * sin(el_angle) + input_q * cos(el_angle));

end

== matlab function motor_simulink/Subsystem1/mid_point_svpwm ==
  data: Ualpha input; Ta output; Ubeta input; Udc input; Tb output; Tc output; Ta_D output; Tb_D output; Tc_D output
function [Ta,Tb,Tc,Ta_D,Tb_D,Tc_D] = fcn(Ualpha,Ubeta,Udc)
Tcm1 = 0;
Tcm2 = 0;
Tcm3 = 0;

Ta=0;
Tb=0;
Tc=0;
Ta_D=0;
Tb_D=0;
Tc_D=0;

Duty_Tcm1 = 0;
Duty_Tcm2 = 0;
Duty_Tcm3 = 0;


Vmax_pu=0;
Vmin_pu=0;
Vcom_pu=0;

Valpha_pu = Ualpha/Udc;
Vbeta_pu = Ubeta/Udc;
    
Va_tmp = 0.5 * Valpha_pu;
Vb_tmp = 0.8660254038 * Vbeta_pu;  %  sqrt(3) / 2

Va_pu = Valpha_pu;
Vb_pu = -Va_tmp + Vb_tmp;                        
Vc_pu = -Va_tmp - Vb_tmp;                        

if(Va_pu > Vb_pu)
    Vmax_pu = Va_pu;
    Vmin_pu = Vb_pu;
end

if(Va_pu <= Vb_pu)
    Vmax_pu = Vb_pu;
    Vmin_pu = Va_pu;
end

if(Vc_pu > Vmax_pu)
    Vmax_pu = Vc_pu;
end
if(Vc_pu < Vmin_pu)
    Vmin_pu = Vc_pu;
end

Vcom_pu = 0.5 * (Vmax_pu + Vmin_pu);            
    
Tcm1 = (Va_pu - Vcom_pu);
Tcm2 = (Vb_pu - Vcom_pu);
Tcm3 = (Vc_pu - Vcom_pu);

if(Tcm1 > 0.5)
    Tcm1 = 0.5;
end
if(Tcm1 < -0.5)
    Tcm1 = -0.5;
end


if(Tcm2 > 0.5)
    Tcm2 = 0.5;
end
if(Tcm2 < -0.5)
    Tcm2 = -0.5;
end


if(Tcm3 > 0.5)
    Tcm3 = 0.5;
end
if(Tcm3 < -0.5)
    Tcm3 = -0.5;
end

Duty_Tcm1 = Tcm1 + 0.5;
Duty_Tcm2 = Tcm2 + 0.5;
Duty_Tcm3 = Tcm3 + 0.5;


Ta=Duty_Tcm1 * 2880;
Tb=Duty_Tcm2 * 2880;
Tc=Duty_Tcm3 * 2880;

Ta_D=Ta-20;
Tb_D=Tb-20;
Tc_D=Tc-20;

if (Ta_D < 0)
    Ta_D=0;
end

if (Tb_D < 0)
    Tb_D=0;
end

if (Tc_D < 0)
    Tc_D=0;
end

%Va = Duty_Tcm1 * Udc;
%Vb = Duty_Tcm2 * Udc;
%Vc = Duty_Tcm3 * Udc;

%Va = Duty_Tcm1;
%Vb = Duty_Tcm2;
%Vc = Duty_Tcm3;

end

== matlab function motor_simulink/Subsystem1/mid_point_svpwm1 ==
  data: Ualpha input; Duty_Tcm1 output; Ubeta input; Udc input; Duty_Tcm2 output; Duty_Tcm3 output
function [Duty_Tcm1,Duty_Tcm2,Duty_Tcm3] = fcn(Ualpha,Ubeta,Udc)
Tcm1 = 0;
Tcm2 = 0;
Tcm3 = 0;

Duty_Tcm1 = 0;
Duty_Tcm2 = 0;
Duty_Tcm3 = 0;


Vmax_pu=0;
Vmin_pu=0;
Vcom_pu=0;

Valpha_pu = Ualpha/Udc;
Vbeta_pu = Ubeta/Udc;
	
Va_tmp = 0.5 * Valpha_pu;
Vb_tmp = 0.8660254038 * Vbeta_pu;

Va_pu = Valpha_pu;
Vb_pu = -Va_tmp + Vb_tmp;						
Vc_pu = -Va_tmp - Vb_tmp;						

if(Va_pu > Vb_pu)
    Vmax_pu = Va_pu;
    Vmin_pu = Vb_pu;
end

if(Va_pu <= Vb_pu)
    Vmax_pu = Vb_pu;
    Vmin_pu = Va_pu;
end

if(Vc_pu > Vmax_pu)
    Vmax_pu = Vc_pu;
end
if(Vc_pu < Vmin_pu)
    Vmin_pu = Vc_pu;
end

Vcom_pu = 0.5 * (Vmax_pu + Vmin_pu);			
	
Tcm1 = (Va_pu - Vcom_pu);
Tcm2 = (Vb_pu - Vcom_pu);
Tcm3 = (Vc_pu - Vcom_pu);

if(Tcm1 > 0.5)
    Tcm1 = 0.5;
end
if(Tcm1 < -0.5)
    Tcm1 = -0.5;
end


if(Tcm2 > 0.5)
    Tcm2 = 0.5;
end
if(Tcm2 < -0.5)
    Tcm2 = -0.5;
end


if(Tcm3 > 0.5)
    Tcm3 = 0.5;
end
if(Tcm3 < -0.5)
    Tcm3 = -0.5;
end

Duty_Tcm1 = Tcm1 + 0.5;
Duty_Tcm2 = Tcm2 + 0.5;
Duty_Tcm3 = Tcm3 + 0.5;

== matlab function motor_simulink/Subsystem/Batterworth ==
  data: b0 input; U_dh_DC output; b1 input; b2 input; a1 input; a2 input; U_qh_DC output; Udh input; Uqh input
function [U_dh_DC,U_qh_DC]= fcn(b0,b1,b2,a1,a2,Udh,Uqh)

persistent first_flag
persistent x_0
persistent x_1
persistent x_2
persistent x_3
persistent x_4
persistent x_5
persistent y_1
persistent y_2
persistent y_3
persistent y_4
persistent y_0_d
persistent y_0_q
if isempty(first_flag)
    U_dh_DC=0;
    U_qh_DC=0;
    x_0=0;
    x_1=0;
    x_2=0;
    y_1=0;
    y_2=0;
    x_3=0;
    x_4=0;
    x_5=0;
    y_3=0;
    y_4=0;
    y_0_d=0;
    y_0_q=0;

    first_flag=true;
end

x_2 = x_1;
x_1 = x_0;
x_0 = Udh;

x_5 = x_4;
x_4 = x_3;
x_3 = Uqh;

y_2 = y_1;
y_1 = y_0_d;

y_4 = y_3;
y_3 = y_0_q;


U_dh_DC = b0*x_0 + b1*x_1 + b2*x_2 - a1*y_1 - a2*y_2;
U_qh_DC = b0*x_3 + b1*x_4 + b2*x_5 - a1*y_3 - a2*y_4;

y_0_d = U_dh_DC;
y_0_q = U_qh_DC;

end

== matlab function motor_simulink/Subsystem/MATLAB Function ==
  data: fs input; b0 output; fc input; b1 output; b2 output; a1 output; a2 output
function [b0, b1, b2, a1, a2] = butterworth_2nd(fs, fc)

persistent first_flag
persistent b_0
persistent b_1
persistent b_2
persistent a_1
persistent a_2

if isempty(first_flag)

    Wn = fc / (fs/2);

    [b, a] = butter(2, Wn, 'low');

    b_0 = b(1);
    b_1 = b(2);
    b_2 = b(3);

    a_1 = a(2);
    a_2 = a(3);

    first_flag=true;
end

b0 = b_0;
b1 = b_1;
b2 = b_2;

a1 = a_1;
a2 = a_2;

end

== matlab function motor_simulink/MATLAB Function ==
  data: Ld_output output; Hz input; Lq_output output; A_hi input; U_dh_DC input; U_qh_DC input
function [Ld_output,Lq_output] = Lq_Ld(Hz,A_hi,U_dh_DC,U_qh_DC)

Ld_output = abs(A_hi / (2 * 2 * pi * Hz * U_dh_DC));
Lq_output = abs(A_hi / (2 * 2 * pi * Hz * U_qh_DC));

end

== matlab function motor_simulink/Subsystem3/MATLAB Function ==
  data: origin_pluse input; output output; add_num input
function output  = train_origin(origin_pluse,add_num)

persistent sum_pluse
persistent flag_now
persistent flag_sum

if(isempty(sum_pluse))
    sum_pluse=0;
    flag_now=0;
    flag_sum=0;
end
if (origin_pluse == 1 && flag_now == 0)
    flag_now = 1;
end

if (origin_pluse == 0 && flag_now == 1)
    flag_now = 0;
    flag_sum = 0;
end

if(flag_now == 1 && flag_sum == 0)
    flag_sum = 1;
    sum_pluse = sum_pluse + add_num;
end

output = sum_pluse;
